simulink model "observador"  (R2015a)
settings: Solver=ode45  StartTime=0.0  StopTime=20  RelTol=1e-3
values from neighbouring files (symbols this model uses):
  A = A    [design.m]    (also in init.mat = [2.98564337206 1 0 0 0 -3.00327796547 0 1 0 0 0.709627661926)
  B = B    [design.m]    (also in init.mat = [1 0 0 0 0])
  C = [-0.0746143795197 0.142131862116 0 0 0]    [init.mat]
  D = zeros(1+length(A(:,1)),1)    [design.m]    (also in init.mat = 0)
  H = [C;eye(size(A))]    [design.m]
undefined symbols (not defined in the file or in its folder): M
settings Model: Creator=João  LastModifiedBy=João

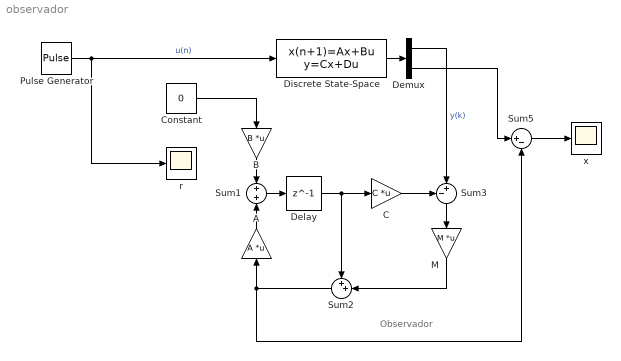
== system observador ==
  note: Observador
  A : Gain  Gain=A  Multiplication=Matrix(K*u) (u vector)
  B : Gain  Gain=B  Multiplication=Matrix(K*u) (u vector)
  C : Gain  Gain=C  Multiplication=Matrix(K*u) (u vector)
  Constant : Constant  Value=0
  Delay : Delay  DelayLength=1  InitialCondition=0  SampleTime=0.02
  Demux : Demux  Outputs=2
  Discrete State-Space : DiscreteStateSpace  A=A  B=B  C=H  D=D  SampleTime=0.02
  M : Gain  Gain=M  Multiplication=Matrix(K*u) (u vector)
  Pulse Generator : DiscretePulseGenerator  PulseType=Time based  Period=20  PhaseDelay=1
  Sum1 : Sum  Inputs=+|+
  Sum2 : Sum  Inputs=++|
  Sum3 : Sum  Inputs=-+|
  Sum5 : Sum  Inputs=|+-
  r : Scope
      settings: SaveName=r_o  SampleInput=on
  x : Scope
      settings: SaveName=x_o  SampleInput=on
  wires:
  Pulse Generator/1 -> Discrete State-Space/1, r/1  "u(n)"
  B/1 -> Sum1/1
  Sum1/1 -> Delay/1
  Sum2/1 -> Sum5/2, A/1
  A/1 -> Sum1/2
  Delay/1 -> C/1, Sum2/1
  C/1 -> Sum3/1
  Sum3/1 -> M/1
  M/1 -> Sum2/2
  Discrete State-Space/1 -> Demux/1
  Demux/2 -> Sum5/1
  Sum5/1 -> x/1
  Demux/1 -> Sum3/2  "y(k)"
  Constant/1 -> B/1
